simulink model "sampleModel1999"  (R2023a)
settings: Solver=VariableStepAuto  StartTime=0.0  StopTime=10.0  RelTol=1e-3
libraries: hdlsllib x4, simulink x3
settings Model: Creator=user1  LastModifiedBy=user1

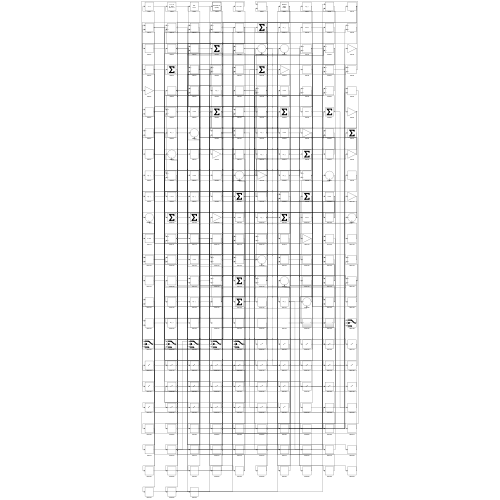
[thumbnail: Simulink's stored preview of the top-level diagram]
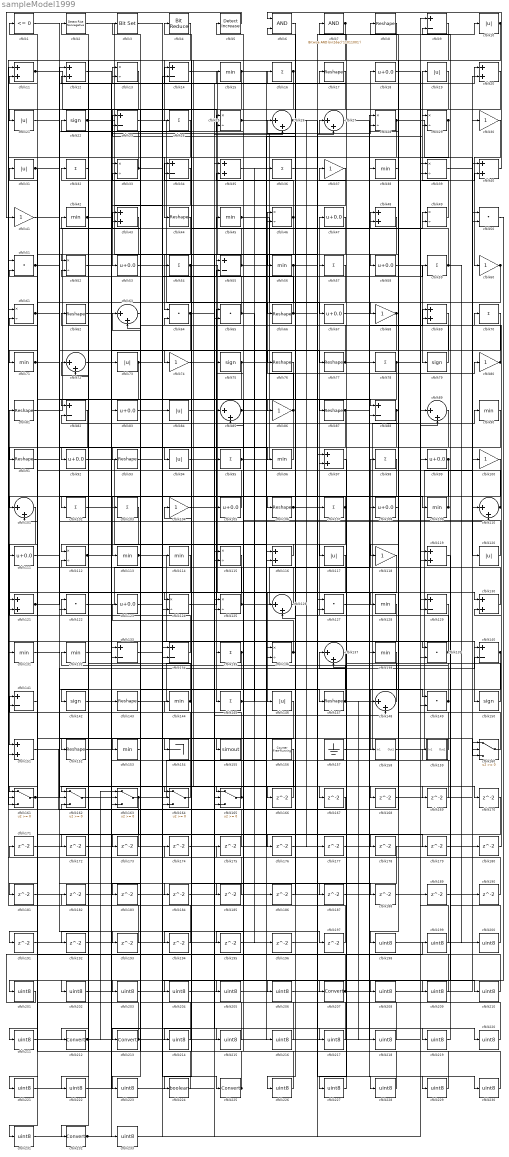
== system sampleModel1999 ==
  cfblk1 : hdlsllib/Logic and Bit Operations/Compare To Zero  relop=<=  OutDataTypeStr=boolean
  cfblk{10,19,21,31,73,84,94,117,120,146} (10 alike) : Abs  SaturateOnIntegerOverflow=off
  cfblk{30,37,41,60,68,74,80,86,100,104,118} (11 alike) : Gain
  cfblk{26..27,63,72,85,89,101,110,126,137,148} (11 alike) : Sum  Inputs=|++
  cfblk{16,24,32,36,54,57,59,70,78,95,98,102..103,107,135,145} (16 alike) : Sum  Inputs=+
  cfblk{18,47,53,58,67,83,92,99,105,108,111,123} (12 alike) : Bias  Bias=0.0  SaturateOnIntegerOverflow=off
  cfblk{8,17,44,62,66,76..77,81,87,91,93,106,143,147,152} (15 alike) : Reshape
  cfblk{15,38,42,45,56,71,90,96,109,113..114,128,131..132,138,144,153} (17 alike) : MinMax
  cfblk{11..12,20,35,40,43,48,69,97,116,119,121,130,151} (14 alike) : Sum
  cfblk{13,25,28..29,33,39,46,49,52,61,112,115,124..125,136} (15 alike) : Product  Inputs=*/  RndMeth=Zero  SaturateOnIntegerOverflow=on
  cfblk{50..51,64..65,122,127,139,149} (8 alike) : DotProduct  OutDataTypeStr=Inherit: Inherit via internal rule
  cfblk{9,14,23,34,55,82,88,129,133..134,140..141} (12 alike) : Sum  Inputs=+-
  cfblk{22,75,79,142,150} (5 alike) : Signum
  cfblk154 : Terminator
  cfblk155 : ToWorkspace  VariableName=simout  SaveFormat=Timeseries  SampleTime=-1
  cfblk156 : hdlsllib/Sources/Counter Free-Running  NumBits=16  tsamp=-1
  cfblk157 : Ground
  cfblk158 : Subsystem
      settings: LibrarySourceBlock=|
      | hdlsllib/Ports &
      | Subsystems/Subsystem
  cfblk159 : Subsystem
      settings: LibrarySourceBlock=|
      | hdlsllib/Ports &
      | Subsystems/Subsystem
  cfblk{160..165} (6 alike) : Switch  SaturateOnIntegerOverflow=off  InputSameDT=off
  cfblk{166..197} (32 alike) : Delay  SampleTime=1
  cfblk{198..206,208..211,214..223,226..231,233} (30 alike) : DataTypeConversion  OutDataTypeStr=uint8  SaturateOnIntegerOverflow=off  RndMeth=Floor
  cfblk2 : hdlsllib/Logic and Bit Operations/Detect Rise Nonnegative  vinit=0  OutDataTypeStr=boolean
  cfblk{207,212..213,225,232} (5 alike) : DataTypeConversion  SaturateOnIntegerOverflow=off  RndMeth=Floor
  cfblk224 : DataTypeConversion  OutDataTypeStr=boolean  SaturateOnIntegerOverflow=off  RndMeth=Floor
  cfblk3 : simulink/Logic and Bit Operations/Bit Set  iBit=0
      settings: LibrarySourceBlock=|
      | hdlsllib/Logic and Bit
      | Operations/Bit Set
  cfblk4 : hdlsllib/Logic and Bit Operations/Bit Reduce  mode=AND
  cfblk5 : simulink/Logic and Bit Operations/Detect Increase  vinit=0.0  OutDataTypeStr=boolean
      settings: LibrarySourceBlock=|
      | hdlsllib/Logic and Bit
      | Operations/Detect
      | Increase
  cfblk6 : Logic  AllPortsSameDT=off  OutDataTypeStr=boolean
  cfblk7 : simulink/Logic and Bit Operations/Bitwise Operator  logicop=AND  UseBitMask=on  BitMask=bin2dec('11011001')  BitMaskRealWorld=Stored Integer
      settings: LibrarySourceBlock=|
      | hdlsllib/Logic and Bit
      | Operations/Bitwise
      | Operator
  wires:
  cfblk134/1 -> cfblk81/1
  cfblk44/1 -> cfblk64/1
  cfblk143/1 -> cfblk22/1
  cfblk8/1 -> cfblk162/1
  cfblk10/1 -> cfblk74/1, cfblk151/2
  cfblk23/1 -> cfblk145/1
  cfblk77/1 -> cfblk42/1, cfblk78/1
  cfblk98/1 -> cfblk113/1
  cfblk151/1 -> cfblk48/1
  cfblk40/1 -> cfblk6/1
  cfblk157/1 -> cfblk90/1
  cfblk15/1 -> cfblk135/1, cfblk140/1, cfblk121/2
  cfblk54/1 -> cfblk128/1, cfblk164/3
  cfblk81/1 -> cfblk38/1
  cfblk26/1 -> cfblk177/1, cfblk220/1
  cfblk125/1 -> cfblk98/1, cfblk11/2, cfblk29/1
  cfblk30/1 -> cfblk60/1
  cfblk139/1 -> cfblk47/1, cfblk23/2
  cfblk116/1 -> cfblk112/1
  cfblk68/1 -> cfblk118/1, cfblk165/2
  cfblk147/1 -> cfblk26/1, cfblk149/1, cfblk218/1, cfblk227/1
  cfblk25/1 -> cfblk88/1, cfblk208/1
  cfblk16/1 -> cfblk21/1, cfblk33/1
  cfblk165/1 -> cfblk141/1, cfblk205/1
  cfblk13/1 -> cfblk53/1
  cfblk18/1 -> cfblk99/1
  cfblk149/1 -> cfblk132/1, cfblk12/2
  cfblk65/1 -> cfblk2/1, cfblk186/1
  cfblk156/1 -> cfblk212/1
  cfblk4/1 -> cfblk24/1
  cfblk3/1 -> cfblk225/1
  cfblk38/1 -> cfblk68/1
  cfblk45/1 -> cfblk67/1, cfblk129/2
  cfblk49/1 -> cfblk19/1
  cfblk5/1 -> cfblk41/1
  cfblk101/1 -> cfblk151/1
  cfblk124/1 -> cfblk65/1
  cfblk75/1 -> cfblk187/1, cfblk202/1
  cfblk150/1 -> cfblk8/1
  cfblk63/1 -> cfblk213/1
  cfblk105/1 -> cfblk51/2
  cfblk91/1 -> cfblk12/1
  cfblk112/1 -> cfblk27/1, cfblk34/2
  cfblk76/1 -> cfblk155/1
  cfblk114/1 -> cfblk232/1
  cfblk158/1(Out1) -> cfblk40/1
  cfblk121/1 -> cfblk25/1, cfblk193/1
  cfblk22/1 -> cfblk105/1, cfblk124/2
  cfblk70/1 -> cfblk94/1
  cfblk118/1 -> cfblk163/3
  cfblk152/1 -> cfblk83/1
  cfblk60/1 -> cfblk125/2, cfblk166/1
  cfblk2/1 -> cfblk107/1
  cfblk92/1 -> cfblk116/2
  cfblk58/1 -> cfblk79/1
  cfblk57/1 -> cfblk65/2
  cfblk96/1 -> cfblk93/1
  cfblk113/1 -> cfblk150/1, cfblk136/1
  cfblk33/1 -> cfblk134/2, cfblk23/1, cfblk206/1
  cfblk73/1 -> cfblk111/1, cfblk136/2
  cfblk122/1 -> cfblk84/1
  cfblk79/1 -> cfblk16/1
  cfblk64/1 -> cfblk17/1, cfblk26/2, cfblk122/2
  cfblk39/1 -> cfblk30/1
  cfblk106/1 -> cfblk20/1, cfblk139/1
  cfblk1/1 -> cfblk87/1
  cfblk27/1 -> cfblk138/1
  cfblk136/1 -> cfblk6/2, cfblk123/1
  cfblk153/1 -> cfblk43/1
  cfblk140/1 -> cfblk158/1(In1), cfblk70/1
  cfblk56/1 -> cfblk91/1, cfblk228/1
  cfblk95/1 -> cfblk18/1, cfblk196/1
  cfblk80/1 -> cfblk32/1, cfblk33/2
  cfblk17/1 -> cfblk52/1
  cfblk48/1 -> cfblk71/1
  cfblk88/1 -> cfblk154/1, cfblk28/2
  cfblk120/1 -> cfblk75/1
  cfblk129/1 -> cfblk153/1
  cfblk71/1 -> cfblk147/1, cfblk176/1
  cfblk32/1 -> cfblk82/1
  cfblk86/1 -> cfblk46/1, cfblk164/2
  cfblk53/1 -> cfblk66/1
  cfblk11/1 -> cfblk55/1, cfblk110/2
  cfblk42/1 -> cfblk103/1, cfblk184/1
  cfblk41/1 -> cfblk130/1
  cfblk61/1 -> cfblk109/1, cfblk179/1, cfblk197/1
  cfblk29/1 -> cfblk148/1, cfblk173/1
  cfblk103/1 -> cfblk152/1
  cfblk109/1 -> cfblk37/1, cfblk85/1
  cfblk159/1(Out1) -> cfblk82/2
  cfblk66/1 -> cfblk4/1, cfblk10/1
  cfblk14/1 -> cfblk56/1
  cfblk117/1 -> cfblk146/1
  cfblk24/1 -> cfblk44/1
  cfblk145/1 -> cfblk46/2, cfblk36/1
  cfblk7/1 -> cfblk106/1, cfblk142/1
  cfblk99/1 -> cfblk194/1, cfblk195/1
  cfblk6/1 -> cfblk76/1
  cfblk126/1 -> cfblk72/1
  cfblk164/1 -> cfblk122/1
  cfblk46/1 -> cfblk124/1, cfblk25/2
  cfblk142/1 -> cfblk165/1
  cfblk163/1 -> cfblk126/1, cfblk181/1
  cfblk51/1 -> cfblk160/3, cfblk49/2
  cfblk148/1 -> cfblk45/1
  cfblk135/1 -> cfblk55/2, cfblk164/1, cfblk224/1
  cfblk128/1 -> cfblk131/1
  cfblk82/1 -> cfblk162/2
  cfblk28/1 -> cfblk120/1, cfblk161/3
  cfblk110/1 -> cfblk14/1, cfblk101/1
  cfblk161/1 -> cfblk140/2, cfblk188/1
  cfblk34/1 -> cfblk133/2
  cfblk62/1 -> cfblk77/1
  cfblk83/1 -> cfblk49/1
  cfblk144/1 -> cfblk62/1, cfblk43/2
  cfblk93/1 -> cfblk59/1
  cfblk36/1 -> cfblk88/2
  cfblk20/1 -> cfblk58/1
  cfblk21/1 -> cfblk13/1
  cfblk87/1 -> cfblk69/1, cfblk161/2
  cfblk162/1 -> cfblk73/1
  cfblk107/1 -> cfblk102/1, cfblk185/1
  cfblk160/1 -> cfblk97/2
  cfblk69/1 -> cfblk92/1
  cfblk55/1 -> cfblk34/1, cfblk29/2
  cfblk72/1 -> cfblk15/1
  cfblk59/1 -> cfblk5/1, cfblk200/1
  cfblk97/1 -> cfblk117/1
  cfblk94/1 -> cfblk57/1
  cfblk102/1 -> cfblk40/2
  cfblk130/1 -> cfblk61/2
  cfblk31/1 -> cfblk96/1, cfblk161/1
  cfblk100/1 -> cfblk207/1
  cfblk85/1 -> cfblk80/1, cfblk28/1
  cfblk74/1 -> cfblk148/2
  cfblk133/1 -> cfblk54/1
  cfblk78/1 -> cfblk129/1, cfblk86/1, cfblk192/1
  cfblk47/1 -> cfblk121/1
  cfblk166/1 -> cfblk64/2
  cfblk111/1 -> cfblk167/1
  cfblk167/1 -> cfblk162/3
  cfblk123/1 -> cfblk168/1
  cfblk168/1 -> cfblk20/2
  cfblk131/1 -> cfblk169/1
  cfblk169/1 -> cfblk133/1
  cfblk84/1 -> cfblk170/1
  cfblk171/1 -> cfblk160/1
  cfblk43/1 -> cfblk172/1
  cfblk172/1 -> cfblk52/2
  cfblk173/1 -> cfblk1/1
  cfblk174/1 -> cfblk116/1
  cfblk175/1 -> cfblk51/1
  cfblk177/1 -> cfblk48/2
  cfblk108/1 -> cfblk178/1
  cfblk179/1 -> cfblk160/2
  cfblk180/1 -> cfblk130/2
  cfblk181/1 -> cfblk39/2
  cfblk182/1 -> cfblk134/1
  cfblk19/1 -> cfblk183/1
  cfblk183/1 -> cfblk13/2
  cfblk184/1 -> cfblk125/1
  cfblk185/1 -> cfblk61/1
  cfblk186/1 -> cfblk126/2
  cfblk187/1 -> cfblk149/2
  cfblk188/1 -> cfblk110/1
  cfblk189/1 -> cfblk69/2
  cfblk190/1 -> cfblk112/2
  cfblk141/1 -> cfblk191/1
  cfblk191/1 -> cfblk97/1
  cfblk192/1 -> cfblk72/2
  cfblk193/1 -> cfblk163/2
  cfblk194/1 -> cfblk11/1
  cfblk195/1 -> cfblk85/2
  cfblk196/1 -> cfblk27/2
  cfblk197/1 -> cfblk101/2
  cfblk9/1 -> cfblk198/1
  cfblk198/1 -> cfblk180/1
  cfblk199/1 -> cfblk9/1
  cfblk200/1 -> cfblk9/2
  cfblk50/1 -> cfblk201/1
  cfblk201/1 -> cfblk199/1
  cfblk202/1 -> cfblk50/1
  cfblk37/1 -> cfblk203/1
  cfblk203/1 -> cfblk50/2
  cfblk89/1 -> cfblk204/1
  cfblk204/1 -> cfblk95/1
  cfblk205/1 -> cfblk89/1
  cfblk206/1 -> cfblk89/2
  cfblk207/1 -> cfblk190/1, cfblk189/1, cfblk141/2
  cfblk208/1 -> cfblk100/1
  cfblk119/1 -> cfblk209/1
  cfblk209/1 -> cfblk7/1
  cfblk176/1 -> cfblk210/1
  cfblk210/1 -> cfblk119/1
  cfblk146/1 -> cfblk211/1
  cfblk211/1 -> cfblk119/2
  cfblk212/1 -> cfblk139/2, cfblk14/2, cfblk163/1
  cfblk213/1 -> cfblk31/1, cfblk108/1
  cfblk178/1 -> cfblk214/1
  cfblk214/1 -> cfblk63/1
  cfblk132/1 -> cfblk215/1
  cfblk215/1 -> cfblk63/2
  cfblk35/1 -> cfblk216/1
  cfblk216/1 -> cfblk174/1
  cfblk12/1 -> cfblk217/1
  cfblk217/1 -> cfblk35/1
  cfblk218/1 -> cfblk35/2
  cfblk104/1 -> cfblk219/1
  cfblk219/1 -> cfblk159/1(In1)
  cfblk220/1 -> cfblk104/1
  cfblk115/1 -> cfblk221/1
  cfblk221/1 -> cfblk143/1
  cfblk170/1 -> cfblk222/1
  cfblk222/1 -> cfblk115/1
  cfblk138/1 -> cfblk223/1
  cfblk223/1 -> cfblk115/2
  cfblk224/1 -> cfblk3/1
  cfblk225/1 -> cfblk182/1, cfblk144/1
  cfblk137/1 -> cfblk226/1
  cfblk226/1 -> cfblk175/1
  cfblk227/1 -> cfblk137/1
  cfblk228/1 -> cfblk137/2
  cfblk127/1 -> cfblk229/1
  cfblk229/1 -> cfblk171/1
  cfblk67/1 -> cfblk230/1
  cfblk230/1 -> cfblk127/1
  cfblk90/1 -> cfblk231/1
  cfblk231/1 -> cfblk127/2
  cfblk232/1 -> cfblk165/3, cfblk39/1
  cfblk52/1 -> cfblk233/1
  cfblk233/1 -> cfblk114/1

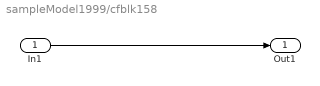
== system sampleModel1999/cfblk158 ==
  In1 : Inport
  Out1 : Outport
  wires:
  In1/1 -> Out1/1

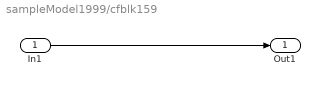
== system sampleModel1999/cfblk159 ==
  In1 : Inport
  Out1 : Outport
  wires:
  In1/1 -> Out1/1
